simulink model "simTwoLinkFTC"  (R2014b)
settings: Solver=ode45  StartTime=0.0  StopTime=tof  FixedStep=dt  MaxStep=dtmax  RelTol=1e-3
values from neighbouring files (symbols this model uses):
  alpha = 1    [robotArmWith2Links.m]    (also in threeLinkFTC.m; twoLinkFTC.m; twoLinkFTCwAdaptive.m)
  Ar = [0 5; -30 -30]    [robotArmWith2Links.m]    (also in threeLinkFTC.m = [0 1; -5 -5]; twoLinkFTC.m = [0 10; -40 -40]; twoLinkFTCwAdaptive.m = [0 5; -250 -250])
  Arm1 = [0 1; -wn^2 -2*ksi*wn]    [robotArmWith2Links.m]    (also in threeLinkFTC.m; twoLinkFTC.m; twoLinkFTCwAdaptive.m)
  As = zeros(nofstates,nofstates)    [threeLinkFTC.m]    (also in twoLinkFDIbasisComparison.m; twoLinkFTC.m; twoLinkFTCwAdaptive.m)
  Brm1 = [0 wn^2]'    [robotArmWith2Links.m]    (also in threeLinkFTC.m; twoLinkFTC.m; twoLinkFTCwAdaptive.m)
  c1 = 0    [robotArmWith2Links.m]    (also in twoLinkFDIbasisComparison.m = 1; twoLinkFTC.m; twoLinkFTCwAdaptive.m)
  c2 = 0    [robotArmWith2Links.m]    (also in twoLinkFDIbasisComparison.m = 1; twoLinkFTC.m; twoLinkFTCwAdaptive.m)
  Dhat0 = zeros(6,1)    [threeLinkFTC.m]    (also in twoLinkFDIbasisComparison.m = zeros(4,1); twoLinkFTC.m = zeros(4,1); twoLinkFTCwAdaptive.m = zeros(4,1))
  Dlimit = 10    [threeLinkFTC.m]    (also in twoLinkFTC.m; twoLinkFTCwAdaptive.m)
  dtFc = 1*dtmax    (= 0.001)    [threeLinkFTC.m]    (also in twoLinkFDIbasisComparison.m; twoLinkFTC.m; twoLinkFTCwAdaptive.m)
  epsilon = 0.5    [robotArmWith2Links.m]    (also in threeLinkFTC.m; twoLinkFTC.m; twoLinkFTCwAdaptive.m)
  epsilontheta = 0.01    [threeLinkFTC.m]    (also in twoLinkFDIbasisComparison.m; twoLinkFTC.m; twoLinkFTCwAdaptive.m)
  faultyArm = 3    [threeLinkFTC.m]    (also in twoLinkFDIbasisComparison.m = 2; twoLinkFTC.m = 2; twoLinkFTCwAdaptive.m = 1)
  FDstart = 0.5    [threeLinkFTC.m]    (also in twoLinkFTC.m; twoLinkFTCwAdaptive.m)
  fmPosition = [0 90 -45]'*pi/180    [threeLinkFTC.m]    (also in twoLinkFTC.m = [90 0]'*pi/180; twoLinkFTCwAdaptive.m = [90 0]'*pi/180)
  g = 9.81    [robotArmWith2Links.m]    (also in threeLinkFTC.m; twoLinkFDIbasisComparison.m; twoLinkFTC.m; twoLinkFTCwAdaptive.m)
  GammaW = 1000    [threeLinkFTC.m]    (also in twoLinkFDIbasisComparison.m; twoLinkFTC.m; twoLinkFTCwAdaptive.m)
  I1 = 8.33e-2    (= 0.0833)    [robotArmWith2Links.m]    (also in threeLinkFTC.m = 0.0833333333333; twoLinkFDIbasisComparison.m = 0.0833333333333; twoLinkFTC.m = 0.0833333333333; twoLinkFTCwAdaptive.m = 0.0833333333333)
  I2 = 8.33e-2    (= 0.0833)    [robotArmWith2Links.m]    (also in threeLinkFTC.m = 0.0833333333333; twoLinkFDIbasisComparison.m = 0.0833333333333; twoLinkFTC.m = 0.0833333333333; twoLinkFTCwAdaptive.m = 0.0833333333333)
  ifault = 2    [threeLinkFTC.m]    (also in twoLinkFDIbasisComparison.m; twoLinkFTC.m; twoLinkFTCwAdaptive.m)
  K1 = 2*wn*ksi    (= 87.9645943005)    [robotArmWith2Links.m]    (also in threeLinkFTC.m = 8.79645943005; twoLinkFTC.m; twoLinkFTCwAdaptive.m = 43.9822971503)
  K2 = wn^2    (= 986.960440109)    [robotArmWith2Links.m]    (also in threeLinkFTC.m = 39.4784176044; twoLinkFTC.m; twoLinkFTCwAdaptive.m)
  Kp = wn^2    (= 157.913670417)    [threeLinkFTC.m]    (also in twoLinkFDIbasisComparison.m = 3947.84176044; twoLinkFTC.m = 3947.84176044; twoLinkFTCwAdaptive.m = 3947.84176044)
  Kv = 2*ksi*wn    (= 17.5929188601)    [threeLinkFTC.m]    (also in twoLinkFDIbasisComparison.m = 125.663706144; twoLinkFTC.m = 125.663706144; twoLinkFTCwAdaptive.m = 125.663706144)
  l1 = 1    [robotArmWith2Links.m]    (also in threeLinkFTC.m; twoLinkFDIbasisComparison.m; twoLinkFTC.m; twoLinkFTCwAdaptive.m)
  l2 = 1    [robotArmWith2Links.m]    (also in threeLinkFTC.m; twoLinkFDIbasisComparison.m; twoLinkFTC.m; twoLinkFTCwAdaptive.m)
  lc1 = l1/2    (= 0.5)    [robotArmWith2Links.m]    (also in threeLinkFTC.m; twoLinkFDIbasisComparison.m; twoLinkFTC.m; twoLinkFTCwAdaptive.m)
  lc2 = l2/2    (= 0.5)    [robotArmWith2Links.m]    (also in threeLinkFTC.m; twoLinkFDIbasisComparison.m; twoLinkFTC.m; twoLinkFTCwAdaptive.m)
  m1 = 1    [robotArmWith2Links.m]    (also in threeLinkFTC.m; twoLinkFDIbasisComparison.m; twoLinkFTC.m; twoLinkFTCwAdaptive.m)
  m2 = 1    [robotArmWith2Links.m]    (also in threeLinkFTC.m; twoLinkFDIbasisComparison.m; twoLinkFTC.m; twoLinkFTCwAdaptive.m)
  nCheby = 4    [threeLinkFTC.m]    (also in twoLinkFDIbasisComparison.m; twoLinkFTC.m; twoLinkFTCwAdaptive.m)
  Ps = lyap(As(4:6,4:6)',Q)    [threeLinkFTC.m]    (also in twoLinkFDIbasisComparison.m = lyap(As(3:4,3:4)',Q); twoLinkFTC.m = lyap(As(3:4,3:4)',Q); twoLinkFTCwAdaptive.m = lyap(As(3:4,3:4)',Q))
  q0 = [80 20]'*pi/180    [robotArmWith2Links.m]    (also in threeLinkFTC.m = [90 0 0]'*pi/180; twoLinkFDIbasisComparison.m = [90 0]'*pi/180; twoLinkFTC.m = [90 0]'*pi/180; twoLinkFTCwAdaptive.m = [90 0]'*pi/180)
  qdot0 = [0 0]'    [robotArmWith2Links.m]    (also in threeLinkFTC.m = [0 0 0]'*pi/180; twoLinkFDIbasisComparison.m = [0 0]'*pi/180; twoLinkFTC.m = [0 0]'*pi/180; twoLinkFTCwAdaptive.m = [0 0]'*pi/180)
  r0 = [0 0]'    [robotArmWith2Links.m]    (also in threeLinkFTC.m; twoLinkFTC.m; twoLinkFTCwAdaptive.m)
  rmax = inf*[50*pi/180 inf]'    [robotArmWith2Links.m]    (also in threeLinkFTC.m; twoLinkFTC.m; twoLinkFTCwAdaptive.m)
  rmin = -rmax    [robotArmWith2Links.m]    (also in threeLinkFTC.m; twoLinkFTC.m; twoLinkFTCwAdaptive.m)
  tfault = 5    [threeLinkFTC.m]    (also in twoLinkFDIbasisComparison.m; twoLinkFTC.m; twoLinkFTCwAdaptive.m = 1)
  visualFlag = 0    [robotArmWith2Links.m]    (also in twoLinkFDIbasisComparison.m; twoLinkFTC.m; twoLinkFTCwAdaptive.m)
  visualizationDataFlag = 1    [robotArmWith2Links.m]    (also in twoLinkFDIbasisComparison.m; twoLinkFTC.m; twoLinkFTCwAdaptive.m)
  W0 = 0    [threeLinkFTC.m]    (also in twoLinkFDIbasisComparison.m; twoLinkFTC.m; twoLinkFTCwAdaptive.m)
  Wbnd = 1000    [threeLinkFTC.m]    (also in twoLinkFDIbasisComparison.m; twoLinkFTC.m; twoLinkFTCwAdaptive.m)
  xhat0 = [q0 ; qdot0]    [threeLinkFTC.m]    (also in twoLinkFDIbasisComparison.m; twoLinkFTC.m; twoLinkFTCwAdaptive.m)
undefined symbols (not defined in the file or in its folder): Intmax, Intmin, twolinkplot
libraries: simulink x6, vrlib x2, dspbuff3 x1
(part 2 of 2)

== system simTwoLinkFTC/System/System Parameters/Energy Calculation ==
  q : Inport
  qdot : Inport  Port=2
  H : Inport  Port=3
  Constant : Constant  Value=l1  VectorParams1D=off
  Constant1 : Constant  Value=l2  VectorParams1D=off
  Demux : Demux  Outputs=2
  Gain : Gain  Gain=1/2
  Gain1 : Gain  Gain=0.5
  Gain5 : Gain  Gain=0.5*m1*g
  Gain6 : Gain  Gain=m2*g
  Math Function : Math  Operator=transpose  SaturateOnIntegerOverflow=on
  Product1 : Product  RndMeth=Zero
  Product3 : Product  RndMeth=Zero
  Product5 : Product  Inputs=3  Multiplication=Matrix(*)  RndMeth=Zero
  Sum of Elements : Sum  Inputs=+
  Sum1 : Sum
  Sum2 : Sum
  Sum3 : Sum
  Terminator4 : Terminator
  Trigonometric Function : Trigonometry
  Trigonometric Function2 : Trigonometry
  U : Outport
  T : Outport  Port=2
  E : Outport  Port=3
  wires:
  [q] -> Trigonometric Function/1, Sum of Elements/1
  Trigonometric Function/1 -> Demux/1
  Demux/1 -> [s1]
  Demux/2 -> Terminator4/1
  Sum of Elements/1 -> Trigonometric Function2/1
  Trigonometric Function2/1 -> [s12]
  [qdot] -> Math Function/1
  Math Function/1 -> Product5/1
  [H] -> Product5/2
  [qdot] -> Product5/3
  Product5/1 -> Gain/1
  [l1sintht1] -> Gain5/1
  Gain/1 -> [T]
  [l1sintht1] -> Sum1/1
  [l2sintht12] -> Gain1/1
  Gain5/1 -> Sum3/1
  Gain6/1 -> Sum3/2
  [T] -> Sum2/1
  [U] -> Sum2/2
  q/1 -> [q]
  qdot/1 -> [qdot]
  Sum2/1 -> E/1  "E"
  [U] -> U/1  "U"
  [T] -> T/1  "T"
  Constant/1 -> Product1/1
  [s1] -> Product1/2
  Product1/1 -> [l1sintht1]
  Constant1/1 -> Product3/1
  [s12] -> Product3/2
  Product3/1 -> [l2sintht12]
  Gain1/1 -> Sum1/2
  Sum1/1 -> Gain6/1
  Sum3/1 -> [U]
  H/1 -> [H]

== system simTwoLinkFTC/System/System Parameters/get Plant Parameters ==
  H : Inport
  C : Inport  Port=2
  G : Inport  Port=3
  qdot : Inport  Port=4
  {1,5,7,11} (4 alike) : Selector  NumberOfDimensions=2  InputPortWidth=3  IndexOptions=Index vector (dialog),Index vector (dialog)  Indices=1,1  OutputSizes=1,1
  12 : Selector  NumberOfDimensions=2  InputPortWidth=3  IndexOptions=Index vector (dialog),Index vector (dialog)  Indices=1,2  OutputSizes=1,1
  2 : Selector  NumberOfDimensions=2  InputPortWidth=3  IndexOptions=Index vector (dialog),Index vector (dialog)  Indices=1,2  OutputSizes=1,1
  {3,6,8,21} (4 alike) : Selector  NumberOfDimensions=2  InputPortWidth=3  IndexOptions=Index vector (dialog),Index vector (dialog)  Indices=2,1  OutputSizes=1,1
  22 : Selector  NumberOfDimensions=2  InputPortWidth=3  IndexOptions=Index vector (dialog),Index vector (dialog)  Indices=2,2  OutputSizes=1,1
  4 : Selector  NumberOfDimensions=2  InputPortWidth=3  IndexOptions=Index vector (dialog),Index vector (dialog)  Indices=2,2  OutputSizes=1,1
  Bus Creator : BusCreator  Inputs=15
  Product5 : Product  Multiplication=Matrix(*)  RndMeth=Zero
  Sum of Elements1 : Sum
  busData : Outport
  wires:
  2/1 -> Bus Creator/9  "C12"
  21/1 -> Bus Creator/6  "H21"
  22/1 -> Bus Creator/7  "H22"
  4/1 -> Bus Creator/11  "C22"
  6/1 -> Bus Creator/13  "G_2"
  1/1 -> Bus Creator/8  "C11"
  5/1 -> Bus Creator/12  "G_1"
  12/1 -> Bus Creator/5  "H12"
  3/1 -> Bus Creator/10  "C21"
  11/1 -> Bus Creator/4  "H11"
  [H] -> 11/1, 12/1, 21/1, 22/1
  [C] -> 1/1, 2/1, 4/1, 3/1
  [G] -> 6/1, 5/1
  [C] -> Product5/1
  [qdot] -> Product5/2
  Product5/1 -> Sum of Elements1/1
  [G] -> Sum of Elements1/2
  Sum of Elements1/1 -> 7/1, 8/1
  7/1 -> Bus Creator/14  "phi1"
  8/1 -> Bus Creator/15  "phi2"
  [G] -> Bus Creator/3
  Bus Creator/1 -> busData/1
  [C] -> Bus Creator/2
  [H] -> Bus Creator/1
  H/1 -> [H]  "H"
  C/1 -> [C]  "C"
  G/1 -> [G]  "G"
  qdot/1 -> [qdot]

== system simTwoLinkFTC/System/System Parameters/getC ==
  s2 : Inport
  q1dot : Inport  Port=2
  q2dot : Inport  Port=3
  m2 : Inport  Port=4
  Add : Sum
  Constant2 : Constant  Value=c2  VectorParams1D=off
  Constant3 : Constant  Value=c1  VectorParams1D=off
  Gain4 : Gain  Gain=l1*lc2
  Gain6 : Gain  Gain=-1
  Gain7 : Gain  Gain=-1
  Matrix Concatenate : Concatenate  Mode=Multidimensional array  ConcatenateDimension=2
  Matrix Concatenate1 : Concatenate  Mode=Multidimensional array  ConcatenateDimension=2
  Matrix Concatenate2 : Concatenate  Mode=Multidimensional array
  Product{,8..10} (4 alike) : Product  RndMeth=Zero
  Sum4 : Sum
  C : Outport
  wires:
  s2/1 -> [s2]
  q1dot/1 -> [q1dot]
  q2dot/1 -> [q2dot]
  [C] -> C/1
  [m2] -> Gain4/1
  Gain4/1 -> Product/1
  [s2] -> Product/2
  Product/1 -> [h]
  [h] -> Gain6/1
  [h] -> Gain7/1
  Sum4/1 -> Product10/1
  Gain7/1 -> Product10/2
  Product10/1 -> [C12]
  [q2dot] -> Sum4/2
  Constant2/1 -> [C22]
  [h] -> Product8/2
  [q1dot] -> Product8/1
  Product8/1 -> [C21]
  Gain6/1 -> Product9/2
  [q2dot] -> Product9/1
  [q1dot] -> Sum4/1
  Matrix Concatenate2/1 -> [C]
  [C22] -> Matrix Concatenate1/2
  [C21] -> Matrix Concatenate1/1
  Matrix Concatenate1/1 -> Matrix Concatenate2/2
  Matrix Concatenate/1 -> Matrix Concatenate2/1
  [C12] -> Matrix Concatenate/2
  [C11] -> Matrix Concatenate/1
  Product9/1 -> Add/1
  Constant3/1 -> Add/2
  Add/1 -> [C11]
  m2/1 -> [m2]

== system simTwoLinkFTC/System/System Parameters/getG ==
  c1 : Inport
  c12 : Inport  Port=2
  m1 : Inport  Port=3
  m2 : Inport  Port=4
  Add1 : Sum
  Add2 : Sum
  Gain10 : Gain  Gain=lc2
  Gain11 : Gain  Gain=g
  Gain5 : Gain  Gain=lc1
  Gain6 : Gain  Gain=l1
  Gain7 : Gain  Gain=g
  Gain8 : Gain  Gain=lc2
  Gain9 : Gain  Gain=g
  Matrix Concatenate2 : Concatenate  Mode=Multidimensional array
  Product1 : Product  RndMeth=Zero
  Product2 : Product  RndMeth=Zero
  Product3 : Product  RndMeth=Zero
  G : Outport
  wires:
  c12/1 -> [c12]
  c1/1 -> [c1]
  Matrix Concatenate2/1 -> G/1
  [G11] -> Matrix Concatenate2/1
  [G21] -> Matrix Concatenate2/2
  [m1] -> Gain5/1
  Gain5/1 -> Add1/1
  [m2] -> Gain6/1
  Gain6/1 -> Add1/2
  Add1/1 -> Gain7/1
  Gain7/1 -> Product1/1
  [c1] -> Product1/2
  [m2] -> Gain8/1
  Gain8/1 -> Gain9/1
  Gain9/1 -> Product2/1
  [c12] -> Product2/2
  Product1/1 -> Add2/1
  Product2/1 -> Add2/2
  Add2/1 -> [G11]
  [m2] -> Gain10/1
  Gain10/1 -> Gain11/1
  Gain11/1 -> Product3/1
  [c12] -> Product3/2
  Product3/1 -> [G21]
  m1/1 -> [m1]
  m2/1 -> [m2]

== system simTwoLinkFTC/System/System Parameters/getH ==
  c2 : Inport
  m1 : Inport  Port=2
  m2 : Inport  Port=3
  I1 : Inport  Port=4
  I2 : Inport  Port=5
  Gain : Gain  Gain=2
  Gain1 : Gain  Gain=lc2^2
  Gain4 : Gain  Gain=l1*lc2
  Gain5 : Gain  Gain=lc1^2
  Gain6 : Gain  Gain=l1^2+lc2^2
  Gain7 : Gain  Gain=lc2^2
  Matrix Concatenate : Concatenate  Mode=Multidimensional array  ConcatenateDimension=2
  Matrix Concatenate1 : Concatenate  Mode=Multidimensional array  ConcatenateDimension=2
  Matrix Concatenate2 : Concatenate  Mode=Multidimensional array
  Product : Product  RndMeth=Zero
  Sum : Sum  Inputs=+++++
  Sum1 : Sum  Inputs=+++
  Sum2 : Sum
  H : Outport
  wires:
  [H11] -> Matrix Concatenate/1
  [H12] -> Matrix Concatenate/2
  Matrix Concatenate/1 -> Matrix Concatenate2/1
  Matrix Concatenate1/1 -> Matrix Concatenate2/2
  [H21] -> Matrix Concatenate1/1
  [H22] -> Matrix Concatenate1/2
  Matrix Concatenate2/1 -> H/1
  c2/1 -> [c2]
  Sum/1 -> [H11]
  Sum1/1 -> [H12], [H21]
  [m2] -> Gain4/1
  Gain4/1 -> Product/1
  [c2] -> Product/2
  Product/1 -> [a]
  [m1] -> Gain5/1
  [m2] -> Gain6/1
  [I1] -> Sum/1
  [I2] -> Sum/2
  Gain5/1 -> Sum/3
  [a] -> Gain/1
  Gain6/1 -> Sum/4
  Gain/1 -> Sum/5
  [m2] -> Gain7/1
  [I2] -> Sum1/1
  Gain7/1 -> Sum1/2
  [a] -> Sum1/3
  [m2] -> Gain1/1
  [I2] -> Sum2/1
  Gain1/1 -> Sum2/2
  Sum2/1 -> [H22]
  m1/1 -> [m1]
  m2/1 -> [m2]
  I1/1 -> [I1]
  I2/1 -> [I2]

== system simTwoLinkFTC/System/System Parameters/getH1 ==
  c2 : Inport
  m1 : Inport  Port=2
  m2 : Inport  Port=3
  I1 : Inport  Port=4
  I2 : Inport  Port=5
  Gain : Gain  Gain=2
  Gain1 : Gain  Gain=lc2^2
  Gain4 : Gain  Gain=l1*lc2
  Gain5 : Gain  Gain=lc1^2
  Gain6 : Gain  Gain=l1^2+lc2^2
  Gain7 : Gain  Gain=lc2^2
  Matrix Concatenate : Concatenate  Mode=Multidimensional array  ConcatenateDimension=2
  Matrix Concatenate1 : Concatenate  Mode=Multidimensional array  ConcatenateDimension=2
  Matrix Concatenate2 : Concatenate  Mode=Multidimensional array
  Product : Product  RndMeth=Zero
  Sum : Sum  Inputs=+++++
  Sum1 : Sum  Inputs=+++
  Sum2 : Sum
  H : Outport
  wires:
  [H11] -> Matrix Concatenate/1
  [H12] -> Matrix Concatenate/2
  Matrix Concatenate/1 -> Matrix Concatenate2/1
  Matrix Concatenate1/1 -> Matrix Concatenate2/2
  [H21] -> Matrix Concatenate1/1
  [H22] -> Matrix Concatenate1/2
  Matrix Concatenate2/1 -> H/1
  c2/1 -> [c2]
  Sum/1 -> [H11]
  Sum1/1 -> [H12], [H21]
  [m2] -> Gain4/1
  Gain4/1 -> Product/1
  [c2] -> Product/2
  Product/1 -> [a]
  [m1] -> Gain5/1
  [m2] -> Gain6/1
  [I1] -> Sum/1
  [I2] -> Sum/2
  Gain5/1 -> Sum/3
  [a] -> Gain/1
  Gain6/1 -> Sum/4
  Gain/1 -> Sum/5
  [m2] -> Gain7/1
  [I2] -> Sum1/1
  Gain7/1 -> Sum1/2
  [a] -> Sum1/3
  [m2] -> Gain1/1
  [I2] -> Sum2/1
  Gain1/1 -> Sum2/2
  Sum2/1 -> [H22]
  m1/1 -> [m1]
  m2/1 -> [m2]
  I1/1 -> [I1]
  I2/1 -> [I2]

== system simTwoLinkFTC/System/System Parameters/getMass ==
  Constant : Constant  Value=m1
  Constant1 : Constant  Value=m2
  Constant5 : Constant  Value=I1
  Constant6 : Constant  Value=I2
  m1 : Outport
  m2 : Outport  Port=2
  I1 : Outport  Port=3
  I2 : Outport  Port=4
  wires:
  [m1] -> m1/1  "m1"
  [m2] -> m2/1  "m2"
  [I1] -> I1/1  "I1"
  [I2] -> I2/1  "I2"
  Constant5/1 -> [I1]
  Constant/1 -> [m1]
  Constant1/1 -> [m2]
  Constant6/1 -> [I2]

== system simTwoLinkFTC/Controller/Disturbance Estimator/getDisturbance/Chebyshev Basis Functions ==
  x : Inport
  tau : Inport  Port=2
  Chebyshev Polynomail Value Calculation : Subsystem  TreatAsAtomicUnit=on
  Demux : Demux
  Mux : Mux
  Reshape1 : Reshape  OutputDimensionality=Column vector (2-D)
  Reshape2 : Reshape  OutputDimensionality=Column vector (2-D)
  Terminator1 : Terminator
  Tn : Outport
  wires:
  [Tn] -> Tn/1
  [z] -> Chebyshev Polynomail Value Calculation/1(x)
  Chebyshev Polynomail Value Calculation/1(chebyPol) -> Reshape2/1
  Reshape2/1 -> [Tn]
  tau/1 -> Terminator1/1
  x/1 -> [x]
  [x] -> Demux/1
  Demux/1 -> [q1]
  Demux/2 -> [q2]
  Demux/3 -> [q1dot]
  Demux/4 -> [q2dot]
  Mux/1 -> Reshape1/1
  Reshape1/1 -> [z]
  [q1] -> Mux/1
  [q2] -> Mux/2
  [q1dot] -> Mux/3
  [q2dot] -> Mux/4

== system simTwoLinkFTC/Controller/Disturbance Estimator/getDisturbance/Custom Basis Functions ==
  x : Inport
  tau : Inport  Port=2
  Add : Sum
  Constant : Constant
  Demux : Demux
  Math Function : Math  Operator=square  SaturateOnIntegerOverflow=on
  Math Function1 : Math  Operator=square  SaturateOnIntegerOverflow=on
  Mux : Mux  Inputs=7
  Product{1..4} (4 alike) : Product  RndMeth=Zero
  Reshape : Reshape  OutputDimensionality=Column vector (2-D)
  Terminator1 : Terminator
  Trigonometric Function : Trigonometry  Operator=cos
  Trigonometric Function1 : Trigonometry  Operator=cos
  Trigonometric Function{2..5} (4 alike) : Trigonometry
  psiz : Outport
  wires:
  [psiz] -> psiz/1
  Constant/1 -> Mux/1
  Mux/1 -> Reshape/1
  Reshape/1 -> [psiz]
  tau/1 -> Terminator1/1
  x/1 -> [x]
  [x] -> Demux/1
  Demux/1 -> [q1]
  Demux/2 -> [q2]
  Demux/3 -> [q1dot]
  Demux/4 -> [q2dot]
  [q1] -> Trigonometric Function/1
  Trigonometric Function/1 -> Mux/2
  [q1] -> Add/1
  [q2] -> Add/2
  Add/1 -> Trigonometric Function1/1
  Trigonometric Function1/1 -> Mux/3
  [q2] -> Trigonometric Function2/1
  Trigonometric Function2/1 -> Product1/1
  [q1dot] -> Product1/2
  Product1/1 -> Mux/4
  [q2] -> Trigonometric Function3/1
  Trigonometric Function3/1 -> Product2/1
  [q2dot] -> Product2/2
  Product2/1 -> Mux/5
  [q2] -> Trigonometric Function4/1
  Trigonometric Function4/1 -> Product3/1
  [q1dot] -> Math Function/1
  Math Function/1 -> Product3/2
  Product3/1 -> Mux/6
  [q2] -> Trigonometric Function5/1
  Trigonometric Function5/1 -> Product4/1
  [q2dot] -> Math Function1/1
  Math Function1/1 -> Product4/2
  Product4/1 -> Mux/7

== system simTwoLinkFTC/Controller/Disturbance Estimator/getDisturbance/getDhat ==
  psiz : Inport
  es : Inport  Port=2
  Bus Creator : BusCreator  Inputs=2
  Math Function : Math  Operator=transpose  SaturateOnIntegerOverflow=on
  Math Function1 : Math  Operator=transpose  SaturateOnIntegerOverflow=on
  Reshape : Reshape  OutputDimensionality=Column vector (2-D)
  Selector : Selector  NumberOfDimensions=2  InputPortWidth=3  IndexOptions=Select all,Index vector (dialog)  Indices=[1 3],1  OutputSizes=1,1
  Selector1 : Selector  NumberOfDimensions=2  InputPortWidth=3  IndexOptions=Select all,Index vector (dialog)  Indices=[1 3],2  OutputSizes=1,1
  Terminator1 : Terminator
  Vector Concatenate : Concatenate
  adaptiveGain : Subsystem  TreatAsAtomicUnit=on
  getW1 : Subsystem
  getW2 : Subsystem
  Dhat : Outport
  wires:
  es/1 -> [es]  "es"
  adaptiveGain/1(Wintegrand) -> [Wint]  "Wint"
  [Dhat] -> Dhat/1  "Dhat"
  psiz/1 -> [psiz]  "psiz"
  [es] -> adaptiveGain/2(es)
  [psiz] -> adaptiveGain/1(psi(z))
  [psiz] -> getW1/2(psiz)
  Selector/1 -> getW1/1(Wint)
  Vector Concatenate/1 -> Reshape/1
  [psiz] -> getW2/2(psiz)
  Selector1/1 -> getW2/1(Wint)
  Reshape/1 -> [Dhat]
  Bus Creator/1 -> Terminator1/1  "W"
  getW2/2(WTpsi) -> Vector Concatenate/2
  getW1/2(WTpsi) -> Vector Concatenate/1
  getW1/1(W) -> Math Function/1
  getW2/1(W) -> Math Function1/1
  [Wint] -> Selector1/1, Selector/1
  Math Function/1 -> Bus Creator/1  "W1"
  Math Function1/1 -> Bus Creator/2  "W2"

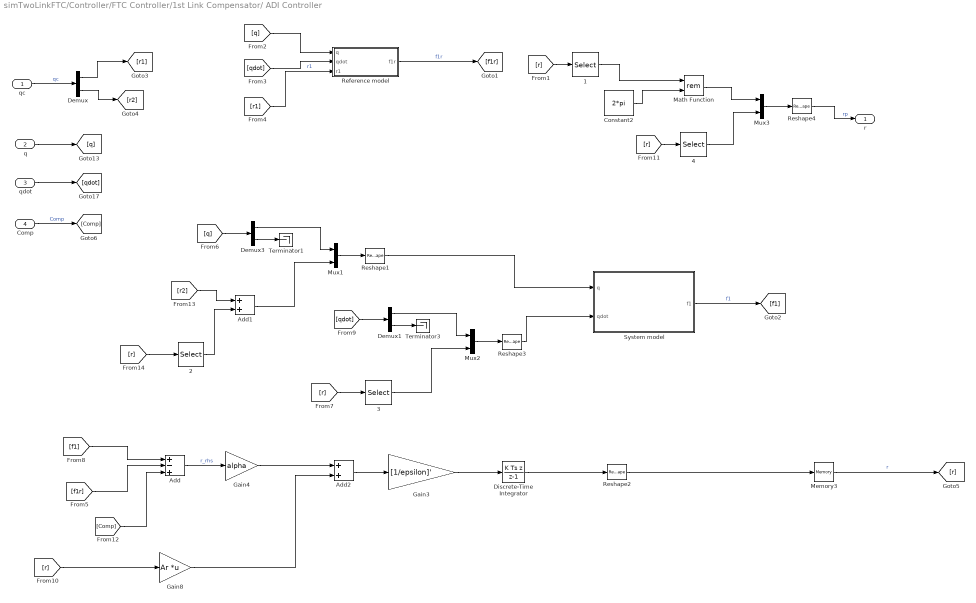
== system simTwoLinkFTC/Controller/FTC Controller/1st Link Compensator/ ADI Controller ==
  qc : Inport
  q : Inport  Port=2
  qdot : Inport  Port=3
  Comp : Inport  Port=4
  1 : Selector  NumberOfDimensions=2  InputPortWidth=3  IndexOptions=Index vector (dialog),Index vector (dialog)  Indices=1,1  OutputSizes=1,1
  2 : Selector  NumberOfDimensions=2  InputPortWidth=3  IndexOptions=Index vector (dialog),Index vector (dialog)  Indices=1,1  OutputSizes=1,1
  3 : Selector  NumberOfDimensions=2  InputPortWidth=3  IndexOptions=Index vector (dialog),Index vector (dialog)  Indices=2,1  OutputSizes=1,1
  4 : Selector  NumberOfDimensions=2  InputPortWidth=3  IndexOptions=Index vector (dialog),Index vector (dialog)  Indices=2,1  OutputSizes=1,1
  Add : Sum  Inputs=+-+
  Add1 : Sum
  Add2 : Sum
  Constant2 : Constant  Value=2*pi
  Demux : Demux  Outputs=2
  Demux1 : Demux  Outputs=2
  Demux3 : Demux  Outputs=2
  Discrete-Time Integrator : DiscreteIntegrator  IntegratorMethod=Integration: Backward Euler  InitialCondition=r0  InitialConditionSetting=State (most efficient)  SampleTime=-1  LimitOutput=on  UpperSaturationLimit=rmax  LowerSaturationLimit=rmin
  Gain3 : Gain  Gain=[1/epsilon]'
  Gain4 : Gain  Gain=alpha
  Gain8 : Gain  Gain=Ar  Multiplication=Matrix(K*u)
  Math Function : Math  Operator=rem  SaturateOnIntegerOverflow=on
  Memory3 : Memory  X0=r0  InheritSampleTime=on  LinearizeMemory=on  LinearizeAsDelay=on
  Mux1 : Mux  Inputs=2
  Mux2 : Mux  Inputs=2
  Mux3 : Mux  Inputs=2
  Reference model : Subsystem  TreatAsAtomicUnit=on
  Reshape{1..4} (4 alike) : Reshape  OutputDimensionality=Column vector (2-D)
  System model : Subsystem  TreatAsAtomicUnit=on
  Terminator1 : Terminator
  Terminator3 : Terminator
  r : Outport
  wires:
  qc/1 -> Demux/1  "qc"
  Add/1 -> Gain4/1  "r_rhs"
  [f1] -> Add/1
  [f1r] -> Add/2
  Gain4/1 -> Add2/1
  Add2/1 -> Gain3/1
  q/1 -> [q]
  qdot/1 -> [qdot]
  [qdot] -> Reference model/2(qdot)
  [q] -> Reference model/1(q)
  [r1] -> Reference model/3(r1)  "r1"
  Reference model/1(f1r) -> [f1r]  "f1r"
  System model/1(f1) -> [f1]  "f1"
  Gain8/1 -> Add2/2
  Reshape3/1 -> System model/2(qdot)
  Demux3/1 -> Mux1/1
  Mux1/1 -> Reshape1/1
  Reshape1/1 -> System model/1(q)
  [q] -> Demux3/1
  Demux3/2 -> Terminator1/1
  [r2] -> Add1/1
  Add1/1 -> Mux1/2
  Memory3/1 -> [r]  "r"
  Constant2/1 -> Math Function/2
  [r] -> 1/1
  Gain3/1 -> Discrete-Time Integrator/1
  Discrete-Time Integrator/1 -> Reshape2/1
  Demux/1 -> [r1]
  Demux/2 -> [r2]
  [r] -> 2/1
  2/1 -> Add1/2
  Demux1/1 -> Mux2/1
  Mux2/1 -> Reshape3/1
  [qdot] -> Demux1/1
  Demux1/2 -> Terminator3/1
  3/1 -> Mux2/2
  [r] -> 3/1
  1/1 -> Math Function/1
  [r] -> Gain8/1
  Mux3/1 -> Reshape4/1
  Reshape4/1 -> r/1  "rp"
  [r] -> 4/1
  Comp/1 -> [Comp]  "Comp"
  [Comp] -> Add/3
  Math Function/1 -> Mux3/1
  4/1 -> Mux3/2
  Reshape2/1 -> Memory3/1

== system simTwoLinkFTC/Controller/FTC Controller/1st Link Compensator/Partial FBL q2 Controller ==
  qc : Inport
  qcdot : Inport  Port=2
  q : Inport  Port=3
  qdot : Inport  Port=4
  H : Inport  Port=5
  C : Inport  Port=6
  G : Inport  Port=7
  Collocated q2 Controller : Subsystem  TreatAsAtomicUnit=on
  Demux{,1..3} (4 alike) : Demux  Outputs=2
  Terminator{1..4} (4 alike) : Terminator
  Torque calculation : Subsystem  TreatAsAtomicUnit=on
  tau : Outport
  v : Outport  Port=2
  wires:
  [q] -> Collocated q2 Controller/3(q)
  Collocated q2 Controller/1(v) -> [v]  "v"
  C/1 -> [C]
  H/1 -> [H]
  qc/1 -> Demux/1
  Demux/1 -> Terminator2/1
  Demux/2 -> [r]
  G/1 -> [G]
  Torque calculation/1(tau) -> [tau]
  [v] -> Torque calculation/1(v)
  [H] -> Torque calculation/2(H)
  [C] -> Torque calculation/3(C)
  [G] -> Torque calculation/4(G)
  [r] -> Collocated q2 Controller/1(r)
  q/1 -> Demux1/1
  Demux1/1 -> Terminator1/1
  Demux1/2 -> [q]
  [qdot] -> Torque calculation/5(qdot)
  qdot/1 -> [qdot]
  [qdot] -> Demux2/1
  Demux2/2 -> Collocated q2 Controller/4(qdot)
  Demux2/1 -> Terminator3/1
  [v] -> v/1
  qcdot/1 -> Demux3/1
  Demux3/1 -> Terminator4/1
  Demux3/2 -> [rdot]
  [rdot] -> Collocated q2 Controller/2(rdot)
  [tau] -> tau/1

== system simTwoLinkFTC/Controller/Disturbance Estimator/getDisturbance/Chebyshev Basis Functions/Chebyshev Polynomail Value Calculation ==
  x : Inport
  Delay Line : dspbuff3/Delay Line  siz=nCheby  ic=zeros(nCheby,1)  directfeed=on  enable_output=off  hold_output=off  TreatMby1Signals=M channels (this choice will be removed - see release notes)
  For Iterator : ForIterator  IterationLimit=nCheby
  Frame Conversion : FrameConversion  OutFrame=Sample-based
  If : If  IfExpression=u1 > 2
  If Action Subsystem : Subsystem  TreatAsAtomicUnit=on
  If Action Subsystem1 : Subsystem  TreatAsAtomicUnit=on
  Memory : Memory  InheritSampleTime=on  LinearizeMemory=on  LinearizeAsDelay=on
  Merge : Merge
  Reshape : Reshape  OutputDimensionality=Column vector (2-D)
  chebyPol : Outport
  wires:
  For Iterator/1 -> [N]
  x/1 -> [x]
  [N] -> If/1
  If/1 -> If Action Subsystem/Action
  If/2 -> If Action Subsystem1/Action
  [N] -> If Action Subsystem1/2(N)
  [x] -> If Action Subsystem1/1(x)
  [x] -> If Action Subsystem/1(x)
  If Action Subsystem/1(polyval) -> Merge/1
  If Action Subsystem1/1(polval) -> Merge/2
  Merge/1 -> [polyval]
  [polyval] -> Delay Line/1
  Delay Line/1 -> Frame Conversion/1
  Reshape/1 -> [polyvals]
  [polyvals] -> Memory/1
  [polyvals] -> chebyPol/1  "chebyPol"
  Frame Conversion/1 -> Reshape/1
  Memory/1 -> If Action Subsystem/2(polyvals)

== system simTwoLinkFTC/Controller/Disturbance Estimator/getDisturbance/getDhat/adaptiveGain ==
  psi(z) : Inport
  es : Inport  Port=2
  Gain1 : Gain  Gain=-1
  Math Function : Math  Operator=transpose  SaturateOnIntegerOverflow=on
  P : Constant  Value=Ps  VectorParams1D=off
  Product1 : Product  Multiplication=Matrix(*)  RndMeth=Zero
  Product3 : Product  Multiplication=Matrix(*)  RndMeth=Zero
  Wintegrand : Outport
  wires:
  Product1/1 -> Product3/2
  psi(z)/1 -> Product3/1
  Gain1/1 -> Wintegrand/1
  es/1 -> Math Function/1
  Math Function/1 -> Product1/1
  P/1 -> Product1/2
  Product3/1 -> Gain1/1

== system simTwoLinkFTC/Controller/Disturbance Estimator/getDisturbance/getDhat/getW1 ==
  Wint : Inport
  psiz : Inport  Port=2
  Constant : Constant  Value=Wbnd  VectorParams1D=off
  Constant1 : Constant  Value=epsilontheta
  Discrete-Time Integrator : DiscreteIntegrator  IntegratorMethod=Integration: Trapezoidal  InitialCondition=W0  SampleTime=-1  LimitOutput=on  UpperSaturationLimit=Wbnd  LowerSaturationLimit=-Wbnd
  Gain : Gain  Gain=GammaW
  Math Function : Math  Operator=transpose  SaturateOnIntegerOverflow=on
  Memory4 : Memory  X0=W0  InheritSampleTime=on  LinearizeMemory=on  LinearizeAsDelay=on
  Product : Product  Multiplication=Matrix(*)  RndMeth=Zero
  Projection : Subsystem  TreatAsAtomicUnit=on
  W : Outport
  WTpsi : Outport  Port=2
  wires:
  [WTpsi] -> WTpsi/1
  [Wint] -> Projection/2(y)
  Math Function/1 -> Product/1
  [psiz] -> Product/2
  Discrete-Time Integrator/1 -> Math Function/1, [W], Memory4/1
  Gain/1 -> Discrete-Time Integrator/1
  Projection/1(Proj) -> Gain/1  "WintProj"
  Memory4/1 -> Projection/1(theta)
  Constant/1 -> Projection/3(Thetamax)
  Constant1/1 -> Projection/4(epsilontheta)
  [W] -> W/1
  Wint/1 -> [Wint]
  psiz/1 -> [psiz]
  Product/1 -> [WTpsi]  "WTpsi"

== system simTwoLinkFTC/Controller/Disturbance Estimator/getDisturbance/getDhat/getW2 ==
  Wint : Inport
  psiz : Inport  Port=2
  Constant : Constant  Value=Wbnd  VectorParams1D=off
  Constant1 : Constant  Value=epsilontheta
  Discrete-Time Integrator : DiscreteIntegrator  IntegratorMethod=Integration: Trapezoidal  InitialCondition=W0  SampleTime=-1  LimitOutput=on  UpperSaturationLimit=Wbnd  LowerSaturationLimit=-Wbnd
  Gain : Gain  Gain=GammaW
  Math Function : Math  Operator=transpose  SaturateOnIntegerOverflow=on
  Memory4 : Memory  X0=W0  InheritSampleTime=on  LinearizeMemory=on  LinearizeAsDelay=on
  Product : Product  Multiplication=Matrix(*)  RndMeth=Zero
  Projection : Subsystem  TreatAsAtomicUnit=on
  W : Outport
  WTpsi : Outport  Port=2
  wires:
  Product/1 -> [WTpsi]  "WTpsi"
  psiz/1 -> [psiz]
  Wint/1 -> [Wint]
  [W] -> W/1
  Constant1/1 -> Projection/4(epsilontheta)
  Constant/1 -> Projection/3(Thetamax)
  Memory4/1 -> Projection/1(theta)
  Projection/1(Proj) -> Gain/1  "WintProj"
  Gain/1 -> Discrete-Time Integrator/1
  Discrete-Time Integrator/1 -> Memory4/1, [W], Math Function/1
  [psiz] -> Product/2
  Math Function/1 -> Product/1
  [Wint] -> Projection/2(y)
  [WTpsi] -> WTpsi/1

== system simTwoLinkFTC/Controller/FTC Controller/1st Link Compensator/ ADI Controller/Reference model ==
  q : Inport
  qdot : Inport  Port=2
  r1 : Inport  Port=3
  Add : Sum
  Constant : Constant  Value=Arm1  VectorParams1D=off
  Constant1 : Constant  Value=Brm1  VectorParams1D=off
  Demux2 : Demux  Outputs=2
  Demux3 : Demux  Outputs=2
  Mux : Mux  Inputs=2
  Product1 : Product  Multiplication=Matrix(*)
  Product3 : Product  Multiplication=Matrix(*)
  Reshape : Reshape  OutputDimensionality=Column vector (2-D)
  Terminator4 : Terminator
  Terminator5 : Terminator
  f1r : Outport
  wires:
  qdot/1 -> Demux3/1
  q/1 -> Demux2/1
  Demux3/2 -> [q2dot]
  Demux3/1 -> [q1dot]
  Demux2/2 -> [q2]
  Demux2/1 -> [q1]
  r1/1 -> [r1]
  Constant/1 -> Product3/1
  [f1r] -> f1r/1
  [q2dot] -> Terminator4/1
  [q2] -> Terminator5/1
  [q1dot] -> Mux/2
  [q1] -> Mux/1
  Mux/1 -> Reshape/1
  Reshape/1 -> Product3/2
  Constant1/1 -> Product1/1
  [r1] -> Product1/2
  Product3/1 -> Add/1
  Product1/1 -> Add/2
  Add/1 -> [f1r]

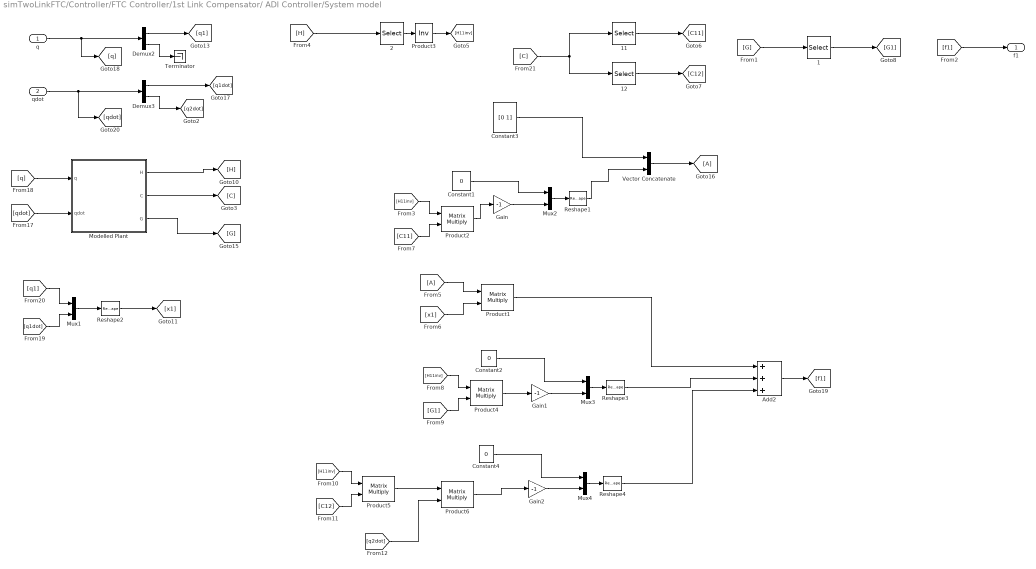
== system simTwoLinkFTC/Controller/FTC Controller/1st Link Compensator/ ADI Controller/System model ==
  q : Inport
  qdot : Inport  Port=2
  1 : Selector  NumberOfDimensions=2  InputPortWidth=3  IndexOptions=Index vector (dialog),Index vector (dialog)  Indices=1,1  OutputSizes=1,1
  11 : Selector  NumberOfDimensions=2  InputPortWidth=3  IndexOptions=Index vector (dialog),Index vector (dialog)  Indices=1,1  OutputSizes=1,1
  12 : Selector  NumberOfDimensions=2  InputPortWidth=3  IndexOptions=Index vector (dialog),Index vector (dialog)  Indices=1,2  OutputSizes=1,1
  2 : Selector  NumberOfDimensions=2  InputPortWidth=3  IndexOptions=Index vector (dialog),Index vector (dialog)  Indices=1,1  OutputSizes=1,1
  Add2 : Sum  Inputs=+++
  Constant1 : Constant  Value=0  VectorParams1D=off
  Constant2 : Constant  Value=0  VectorParams1D=off
  Constant3 : Constant  Value=[0 1]  VectorParams1D=off
  Constant4 : Constant  Value=0  VectorParams1D=off
  Demux2 : Demux  Outputs=2
  Demux3 : Demux  Outputs=2
  Gain : Gain  Gain=-1
  Gain1 : Gain  Gain=-1
  Gain2 : Gain  Gain=-1
  Modelled Plant : Subsystem  TreatAsAtomicUnit=on
  Mux{1..4} (4 alike) : Mux  Inputs=2
  Product{1..2,4..6} (5 alike) : Product  Multiplication=Matrix(*)  RndMeth=Zero
  Product3 : Product  Inputs=/  Multiplication=Matrix(*)  RndMeth=Zero
  Reshape1 : Reshape  OutputDimensionality=Row vector (2-D)
  Reshape2 : Reshape  OutputDimensionality=Column vector (2-D)
  Reshape3 : Reshape  OutputDimensionality=Column vector (2-D)
  Reshape4 : Reshape  OutputDimensionality=Column vector (2-D)
  Terminator : Terminator
  Vector Concatenate : Concatenate  Mode=Multidimensional array
  f1 : Outport
  wires:
  [f1] -> f1/1
  [C] -> 12/1, 11/1
  11/1 -> [C11]
  12/1 -> [C12]
  [G] -> 1/1
  1/1 -> [G1]
  qdot/1 -> [qdot], Demux3/1
  q/1 -> [q], Demux2/1
  Demux3/2 -> [q2dot]
  Demux3/1 -> [q1dot]
  Demux2/2 -> Terminator/1
  Demux2/1 -> [q1]
  [H] -> 2/1
  2/1 -> Product3/1
  Product3/1 -> [H11inv]
  Product1/1 -> Add2/1
  Add2/1 -> [f1]
  [H11inv] -> Product2/1
  [C11] -> Product2/2
  Modelled Plant/1(H) -> [H]
  Modelled Plant/2(C) -> [C]
  Modelled Plant/3(G) -> [G]
  [qdot] -> Modelled Plant/2(qdot)
  [q] -> Modelled Plant/1(q)
  [q1dot] -> Mux1/2
  [q1] -> Mux1/1
  Mux1/1 -> Reshape2/1
  Reshape2/1 -> [x1]
  Product2/1 -> Gain/1
  Constant1/1 -> Mux2/1
  Mux2/1 -> Reshape1/1
  Constant3/1 -> Vector Concatenate/1
  Reshape1/1 -> Vector Concatenate/2
  Vector Concatenate/1 -> [A]
  [A] -> Product1/1
  [x1] -> Product1/2
  [H11inv] -> Product4/1
  [G1] -> Product4/2
  Gain/1 -> Mux2/2
  Product4/1 -> Gain1/1
  Constant2/1 -> Mux3/1
  Mux3/1 -> Reshape3/1
  Gain1/1 -> Mux3/2
  [H11inv] -> Product5/1
  [C12] -> Product5/2
  Constant4/1 -> Mux4/1
  Mux4/1 -> Reshape4/1
  Gain2/1 -> Mux4/2
  Product5/1 -> Product6/1
  [q2dot] -> Product6/2
  Product6/1 -> Gain2/1
  Reshape3/1 -> Add2/2
  Reshape4/1 -> Add2/3

== system simTwoLinkFTC/Controller/FTC Controller/1st Link Compensator/Partial FBL q2 Controller/Collocated q2 Controller ==
  r : Inport
  rdot : Inport  Port=2
  q : Inport  Port=3
  qdot : Inport  Port=4
  Add3 : Sum
  Gain2 : Gain  Gain=-K1
  Gain3 : Gain  Gain=-K2
  sum1 : Sum  Inputs=+-
  sum2 : Sum  Inputs=+-
  v : Outport
  wires:
  Add3/1 -> [v]
  Gain3/1 -> Add3/2
  Gain2/1 -> Add3/1
  [e] -> Gain3/1
  [edot] -> Gain2/1
  qdot/1 -> [qdot]  "qdot"
  q/1 -> [q]  "q"
  [q] -> sum1/1
  [r] -> sum1/2
  sum1/1 -> [e]  "e"
  r/1 -> [r]  "r"
  [v] -> v/1  "v"
  [qdot] -> sum2/1
  [rdot] -> sum2/2
  sum2/1 -> [edot]  "edot"
  rdot/1 -> [rdot]  "rdot"

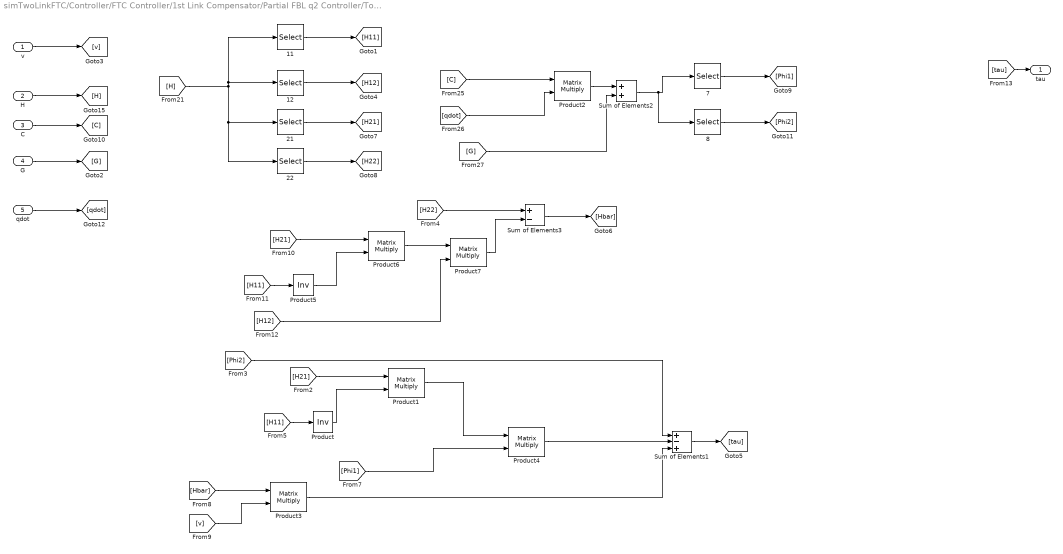
== system simTwoLinkFTC/Controller/FTC Controller/1st Link Compensator/Partial FBL q2 Controller/Torque calculation ==
  v : Inport
  H : Inport  Port=2
  C : Inport  Port=3
  G : Inport  Port=4
  qdot : Inport  Port=5
  11 : Selector  NumberOfDimensions=2  InputPortWidth=3  IndexOptions=Index vector (dialog),Index vector (dialog)  Indices=1,1  OutputSizes=1,1
  12 : Selector  NumberOfDimensions=2  InputPortWidth=3  IndexOptions=Index vector (dialog),Index vector (dialog)  Indices=1,2  OutputSizes=1,1
  21 : Selector  NumberOfDimensions=2  InputPortWidth=3  IndexOptions=Index vector (dialog),Index vector (dialog)  Indices=2,1  OutputSizes=1,1
  22 : Selector  NumberOfDimensions=2  InputPortWidth=3  IndexOptions=Index vector (dialog),Index vector (dialog)  Indices=2,2  OutputSizes=1,1
  7 : Selector  NumberOfDimensions=2  InputPortWidth=3  IndexOptions=Index vector (dialog),Index vector (dialog)  Indices=1,1  OutputSizes=1,1
  8 : Selector  NumberOfDimensions=2  InputPortWidth=3  IndexOptions=Index vector (dialog),Index vector (dialog)  Indices=2,1  OutputSizes=1,1
  Product : Product  Inputs=/  Multiplication=Matrix(*)  RndMeth=Zero
  Product{1..4,6..7} (6 alike) : Product  Multiplication=Matrix(*)  RndMeth=Zero
  Product5 : Product  Inputs=/  Multiplication=Matrix(*)  RndMeth=Zero
  Sum of Elements1 : Sum  Inputs=+-+
  Sum of Elements2 : Sum
  Sum of Elements3 : Sum  Inputs=+-
  tau : Outport
  wires:
  [tau] -> tau/1
  v/1 -> [v]
  [H11] -> Product/1
  [H21] -> Product1/1
  Product/1 -> Product1/2
  Product1/1 -> Product4/1
  [Hbar] -> Product3/1
  [v] -> Product3/2
  Sum of Elements1/1 -> [tau]
  [H11] -> Product5/1
  [H21] -> Product6/1
  Product5/1 -> Product6/2
  Product6/1 -> Product7/1
  [H12] -> Product7/2
  [H22] -> Sum of Elements3/1
  Product7/1 -> Sum of Elements3/2
  Sum of Elements3/1 -> [Hbar]
  [Phi1] -> Product4/2
  [Phi2] -> Sum of Elements1/1
  Product4/1 -> Sum of Elements1/2
  Product3/1 -> Sum of Elements1/3
  C/1 -> [C]
  H/1 -> [H]
  G/1 -> [G]
  [H] -> 11/1, 12/1, 21/1, 22/1
  [C] -> Product2/1
  [qdot] -> Product2/2
  Product2/1 -> Sum of Elements2/1
  [G] -> Sum of Elements2/2
  Sum of Elements2/1 -> 7/1, 8/1
  11/1 -> [H11]
  12/1 -> [H12]
  21/1 -> [H21]
  22/1 -> [H22]
  7/1 -> [Phi1]
  8/1 -> [Phi2]
  qdot/1 -> [qdot]

== system simTwoLinkFTC/Controller/Disturbance Estimator/getDisturbance/Chebyshev Basis Functions/Chebyshev Polynomail Value Calculation/If Action Subsystem ==
  x : Inport
  polyvals : Inport  Port=2
  Action Port : ActionPort  PropagateVarSize=During execution  ActionType=then
  Add : Sum  Inputs=+-
  Constant : Constant  Value=nCheby
  Constant1 : Constant  Value=nCheby-1
  Gain : Gain  Gain=2
  Product : Product  RndMeth=Zero
  Selector : Selector  IndexOptions=Index vector (port)  Indices=[1 3]
  Selector1 : Selector  IndexOptions=Index vector (port)  Indices=[1 3]
  polyval : Outport
  wires:
  x/1 -> [x]
  polyvals/1 -> [polyvals]  "if.polyvals"
  [polyvals] -> Selector/1
  Constant1/1 -> Selector/2
  Selector/1 -> [Tm2]  "Tm2"
  [polyvals] -> Selector1/1
  Constant/1 -> Selector1/2
  Selector1/1 -> [Tm1]  "Tm1"
  [x] -> Product/1
  [Tm1] -> Product/2
  Product/1 -> Gain/1
  Gain/1 -> Add/1
  [Tm2] -> Add/2
  Add/1 -> polyval/1  "if.polyval"

== system simTwoLinkFTC/Controller/Disturbance Estimator/getDisturbance/Chebyshev Basis Functions/Chebyshev Polynomail Value Calculation/If Action Subsystem1 ==
  x : Inport
  N : Inport  Port=2
  Action Port : ActionPort  PropagateVarSize=During execution  ActionType=else
  Bias1 : Bias  Bias=-1
  Data Type Conversion : DataTypeConversion
  Math Function : Math  Operator=pow  OutputSignalType=real  SaturateOnIntegerOverflow=on
  polval : Outport
  wires:
  x/1 -> Math Function/1
  N/1 -> Bias1/1  "else.N"
  Math Function/1 -> polval/1  "else.polyval"
  Data Type Conversion/1 -> Math Function/2
  Bias1/1 -> Data Type Conversion/1

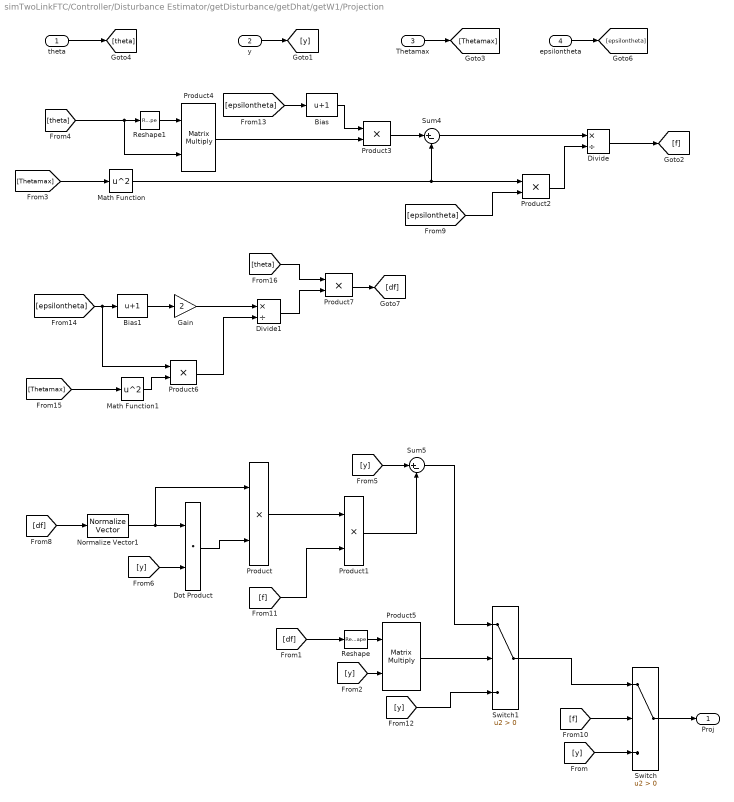
== system simTwoLinkFTC/Controller/Disturbance Estimator/getDisturbance/getDhat/getW1/Projection ==
  theta : Inport
  y : Inport  Port=2
  Thetamax : Inport  Port=3
  epsilontheta : Inport  Port=4
  Bias : Bias  Bias=1
  Bias1 : Bias  Bias=1
  Divide : Product  Inputs=*/
  Divide1 : Product  Inputs=*/
  Dot Product : DotProduct  InputSameDT=on  OutDataTypeStr=Inherit: Inherit via internal rule
  Gain : Gain  Gain=2
  Math Function : Math  Operator=square  SaturateOnIntegerOverflow=on
  Math Function1 : Math  Operator=square  SaturateOnIntegerOverflow=on
  Normalize Vector1 : vrlib/Utilities/Normalize Vector  maxzero=0
  Product{,1..3,6..7} (6 alike) : Product  RndMeth=Zero
  Product4 : Product  Multiplication=Matrix(*)  RndMeth=Zero
  Product5 : Product  Multiplication=Matrix(*)  RndMeth=Zero
  Reshape : Reshape  OutputDimensionality=Row vector (2-D)
  Reshape1 : Reshape  OutputDimensionality=Row vector (2-D)
  Sum4 : Sum  Inputs=|+-
  Sum5 : Sum  Inputs=|+-
  Switch : Switch  Criteria=u2 > Threshold
  Switch1 : Switch  Criteria=u2 > Threshold
  Proj : Outport
  wires:
  [f] -> Switch/2
  y/1 -> [y]
  Switch/1 -> Proj/1
  Product5/1 -> Switch1/2
  [y] -> Product5/2
  Sum4/1 -> Divide/1
  Math Function/1 -> Sum4/2, Product2/1
  Product4/1 -> Product3/2
  [theta] -> Reshape1/1, Product4/2
  [df] -> Reshape/1
  Reshape/1 -> Product5/1
  Reshape1/1 -> Product4/1
  theta/1 -> [theta]
  [y] -> Switch/3
  Switch1/1 -> Switch/1
  [y] -> Sum5/1
  Product/1 -> Product1/1
  [y] -> Switch1/3
  Product1/1 -> Sum5/2
  Sum5/1 -> Switch1/1
  [f] -> Product1/2
  [df] -> Normalize Vector1/1
  Normalize Vector1/1 -> Dot Product/1, Product/1
  [y] -> Dot Product/2
  Dot Product/1 -> Product/2
  Thetamax/1 -> [Thetamax]
  [Thetamax] -> Math Function/1
  epsilontheta/1 -> [epsilontheta]
  [epsilontheta] -> Product2/2
  Product2/1 -> Divide/2
  Divide/1 -> [f]
  Product3/1 -> Sum4/1
  Bias/1 -> Product3/1
  [epsilontheta] -> Bias/1
  [epsilontheta] -> Bias1/1, Product6/1
  Bias1/1 -> Gain/1
  Gain/1 -> Divide1/1
  [Thetamax] -> Math Function1/1
  Math Function1/1 -> Product6/2
  Product6/1 -> Divide1/2
  Product7/1 -> [df]
  [theta] -> Product7/1
  Divide1/1 -> Product7/2

== system simTwoLinkFTC/Controller/Disturbance Estimator/getDisturbance/getDhat/getW2/Projection ==
  theta : Inport
  y : Inport  Port=2
  Thetamax : Inport  Port=3
  epsilontheta : Inport  Port=4
  Bias : Bias  Bias=1
  Bias1 : Bias  Bias=1
  Divide : Product  Inputs=*/
  Divide1 : Product  Inputs=*/
  Dot Product : DotProduct  InputSameDT=on  OutDataTypeStr=Inherit: Inherit via internal rule
  Gain : Gain  Gain=2
  Math Function : Math  Operator=square  SaturateOnIntegerOverflow=on
  Math Function1 : Math  Operator=square  SaturateOnIntegerOverflow=on
  Normalize Vector1 : vrlib/Utilities/Normalize Vector  maxzero=0
  Product{,1..3,6..7} (6 alike) : Product  RndMeth=Zero
  Product4 : Product  Multiplication=Matrix(*)  RndMeth=Zero
  Product5 : Product  Multiplication=Matrix(*)  RndMeth=Zero
  Reshape : Reshape  OutputDimensionality=Row vector (2-D)
  Reshape1 : Reshape  OutputDimensionality=Row vector (2-D)
  Sum4 : Sum  Inputs=|+-
  Sum5 : Sum  Inputs=|+-
  Switch : Switch  Criteria=u2 > Threshold
  Switch1 : Switch  Criteria=u2 > Threshold
  Proj : Outport
  wires:
  Divide1/1 -> Product7/2
  [theta] -> Product7/1
  Product7/1 -> [df]
  Product6/1 -> Divide1/2
  Math Function1/1 -> Product6/2
  [Thetamax] -> Math Function1/1
  Gain/1 -> Divide1/1
  Bias1/1 -> Gain/1
  [epsilontheta] -> Product6/1, Bias1/1
  [epsilontheta] -> Bias/1
  Bias/1 -> Product3/1
  Product3/1 -> Sum4/1
  Divide/1 -> [f]
  Product2/1 -> Divide/2
  [epsilontheta] -> Product2/2
  epsilontheta/1 -> [epsilontheta]
  [Thetamax] -> Math Function/1
  Thetamax/1 -> [Thetamax]
  Dot Product/1 -> Product/2
  [y] -> Dot Product/2
  Normalize Vector1/1 -> Product/1, Dot Product/1
  [df] -> Normalize Vector1/1
  [f] -> Product1/2
  Sum5/1 -> Switch1/1
  Product1/1 -> Sum5/2
  [y] -> Switch1/3
  Product/1 -> Product1/1
  [y] -> Sum5/1
  Switch1/1 -> Switch/1
  [y] -> Switch/3
  theta/1 -> [theta]
  Reshape1/1 -> Product4/1
  Reshape/1 -> Product5/1
  [df] -> Reshape/1
  [theta] -> Product4/2, Reshape1/1
  Product4/1 -> Product3/2
  Math Function/1 -> Product2/1, Sum4/2
  Sum4/1 -> Divide/1
  [y] -> Product5/2
  Product5/1 -> Switch1/2
  Switch/1 -> Proj/1
  y/1 -> [y]
  [f] -> Switch/2

== system simTwoLinkFTC/Controller/FTC Controller/1st Link Compensator/ ADI Controller/System model/Modelled Plant ==
  q : Inport
  qdot : Inport  Port=2
  Demux : Demux  Outputs=2
  Demux1 : Demux  Outputs=2
  Demux2 : Demux  Outputs=2
  Sum of Elements : Sum  Inputs=+
  Terminator4 : Terminator
  Terminator5 : Terminator
  Terminator6 : Terminator
  Trigonometric Function : Trigonometry
  Trigonometric Function1 : Trigonometry  Operator=cos
  Trigonometric Function2 : Trigonometry
  Trigonometric Function3 : Trigonometry  Operator=cos
  get Plant Parameters : Subsystem
  getC : Subsystem
  getG : Subsystem
  getH : Subsystem
  H : Outport
  C : Outport  Port=2
  G : Outport  Port=3
  wires:
  [c2] -> getH/1(c2)
  [s2] -> getC/1(s2)
  [q1dot] -> getC/2(q1dot)
  [q2dot] -> getC/3(q2dot)
  getH/1(H) -> [H]
  getC/1(C) -> [C]
  [c1] -> getG/1(c1)
  [c12] -> getG/2(c12)
  getG/1(G) -> [G]
  q/1 -> Trigonometric Function/1, Trigonometric Function1/1, Sum of Elements/1
  Trigonometric Function/1 -> Demux/1
  Demux/1 -> Terminator4/1
  Demux/2 -> [s2]
  Demux1/1 -> [c1]
  Demux1/2 -> [c2]
  Trigonometric Function1/1 -> Demux1/1
  Sum of Elements/1 -> Trigonometric Function2/1, Trigonometric Function3/1
  Trigonometric Function2/1 -> Terminator5/1
  qdot/1 -> Demux2/1, [qdot]
  Demux2/1 -> [q1dot]
  Demux2/2 -> [q2dot]
  Trigonometric Function3/1 -> [c12]
  [H] -> H/1
  [C] -> C/1
  [G] -> G/1
  get Plant Parameters/1(busData) -> Terminator6/1  "ModeledSystem"
  [C] -> get Plant Parameters/2(C)
  [H] -> get Plant Parameters/1(H)
  [G] -> get Plant Parameters/3(G)
  [qdot] -> get Plant Parameters/4(qdot)

== system simTwoLinkFTC/Controller/FTC Controller/1st Link Compensator/ ADI Controller/System model/Modelled Plant/get Plant Parameters ==
  H : Inport
  C : Inport  Port=2
  G : Inport  Port=3
  qdot : Inport  Port=4
  {1,5,7,11} (4 alike) : Selector  NumberOfDimensions=2  InputPortWidth=3  IndexOptions=Index vector (dialog),Index vector (dialog)  Indices=1,1  OutputSizes=1,1
  12 : Selector  NumberOfDimensions=2  InputPortWidth=3  IndexOptions=Index vector (dialog),Index vector (dialog)  Indices=1,2  OutputSizes=1,1
  2 : Selector  NumberOfDimensions=2  InputPortWidth=3  IndexOptions=Index vector (dialog),Index vector (dialog)  Indices=1,2  OutputSizes=1,1
  {3,6,8,21} (4 alike) : Selector  NumberOfDimensions=2  InputPortWidth=3  IndexOptions=Index vector (dialog),Index vector (dialog)  Indices=2,1  OutputSizes=1,1
  22 : Selector  NumberOfDimensions=2  InputPortWidth=3  IndexOptions=Index vector (dialog),Index vector (dialog)  Indices=2,2  OutputSizes=1,1
  4 : Selector  NumberOfDimensions=2  InputPortWidth=3  IndexOptions=Index vector (dialog),Index vector (dialog)  Indices=2,2  OutputSizes=1,1
  Bus Creator : BusCreator  Inputs=15
  Product5 : Product  Multiplication=Matrix(*)  RndMeth=Zero
  Sum of Elements1 : Sum
  busData : Outport
  wires:
  2/1 -> Bus Creator/9  "C12"
  21/1 -> Bus Creator/6  "H21"
  22/1 -> Bus Creator/7  "H22"
  4/1 -> Bus Creator/11  "C22"
  6/1 -> Bus Creator/13  "G_2"
  1/1 -> Bus Creator/8  "C11"
  5/1 -> Bus Creator/12  "G_1"
  12/1 -> Bus Creator/5  "H12"
  3/1 -> Bus Creator/10  "C21"
  11/1 -> Bus Creator/4  "H11"
  [H] -> 11/1, 12/1, 21/1, 22/1
  [C] -> 1/1, 2/1, 4/1, 3/1
  [G] -> 6/1, 5/1
  [C] -> Product5/1
  [qdot] -> Product5/2
  Product5/1 -> Sum of Elements1/1
  [G] -> Sum of Elements1/2
  Sum of Elements1/1 -> 7/1, 8/1
  7/1 -> Bus Creator/14  "phi1"
  8/1 -> Bus Creator/15  "phi2"
  [G] -> Bus Creator/3
  Bus Creator/1 -> busData/1
  [C] -> Bus Creator/2
  [H] -> Bus Creator/1
  H/1 -> [H]  "H"
  C/1 -> [C]  "C"
  G/1 -> [G]  "G"
  qdot/1 -> [qdot]

== system simTwoLinkFTC/Controller/FTC Controller/1st Link Compensator/ ADI Controller/System model/Modelled Plant/getC ==
  s2 : Inport
  q1dot : Inport  Port=2
  q2dot : Inport  Port=3
  C calculation 1 : Subsystem
  C calculation 2 : Subsystem
  Gain2 : Gain  Gain=m2*l1*lc2
  Terminator : Terminator
  C : Outport
  wires:
  s2/1 -> [s2]
  q1dot/1 -> [q1dot]
  q2dot/1 -> [q2dot]
  [s2] -> Gain2/1
  Gain2/1 -> [h]
  [q1dot] -> C calculation 1/1(q1dot)
  [q2dot] -> C calculation 1/2(q2dot)
  [h] -> C calculation 1/3(h)
  [q1dot] -> C calculation 2/1(q1dot)
  [q2dot] -> C calculation 2/2(q2dot)
  [h] -> C calculation 2/3(h)
  [C] -> C/1
  C calculation 2/1(C) -> [C]
  C calculation 1/1(C) -> Terminator/1

== system simTwoLinkFTC/Controller/FTC Controller/1st Link Compensator/ ADI Controller/System model/Modelled Plant/getG ==
  c1 : Inport
  c12 : Inport  Port=2
  Add : Sum
  Gain : Gain  Gain=(m1*lc1+m2*l1)*g
  Gain1 : Gain  Gain=m2*g*lc2
  Gain2 : Gain
  Gain4 : Gain  Gain=lc2*m2*g
  Matrix Concatenate2 : Concatenate  Mode=Multidimensional array
  G : Outport
  wires:
  [c12] -> Gain4/1
  Gain4/1 -> [G21]
  c12/1 -> [c12]
  c1/1 -> [c1]
  Matrix Concatenate2/1 -> Gain2/1
  [G11] -> Matrix Concatenate2/1
  [G21] -> Matrix Concatenate2/2
  [c1] -> Gain/1
  Gain/1 -> Add/1
  [c12] -> Gain1/1
  Gain1/1 -> Add/2
  Add/1 -> [G11]
  Gain2/1 -> G/1

== system simTwoLinkFTC/Controller/FTC Controller/1st Link Compensator/ ADI Controller/System model/Modelled Plant/getH ==
  c2 : Inport
  Constant1 : Constant  Value=I1 + I2 + m1*lc1^2 + m2*(l1^2+lc2^2)  VectorParams1D=off
  Constant2 : Constant  Value=I2+m2*lc2^2  VectorParams1D=off
  Constant3 : Constant  Value=I2+m2*lc2^2  VectorParams1D=off
  Gain : Gain  Gain=m2*2*l1*lc2
  Gain1 : Gain  Gain=m2*l1*lc2
  Matrix Concatenate : Concatenate  Mode=Multidimensional array  ConcatenateDimension=2
  Matrix Concatenate1 : Concatenate  Mode=Multidimensional array  ConcatenateDimension=2
  Matrix Concatenate2 : Concatenate  Mode=Multidimensional array
  Sum : Sum
  Sum1 : Sum
  H : Outport
  wires:
  [H11] -> Matrix Concatenate/1
  [H12] -> Matrix Concatenate/2
  Matrix Concatenate/1 -> Matrix Concatenate2/1
  Matrix Concatenate1/1 -> Matrix Concatenate2/2
  [H21] -> Matrix Concatenate1/1
  [H22] -> Matrix Concatenate1/2
  Matrix Concatenate2/1 -> H/1
  c2/1 -> [c2]
  [c2] -> Gain/1
  Gain/1 -> Sum/1
  Constant1/1 -> Sum/2
  Sum/1 -> [H11]
  [c2] -> Gain1/1
  Gain1/1 -> Sum1/1
  Constant2/1 -> Sum1/2
  Sum1/1 -> [H12], [H21]
  Constant3/1 -> [H22]

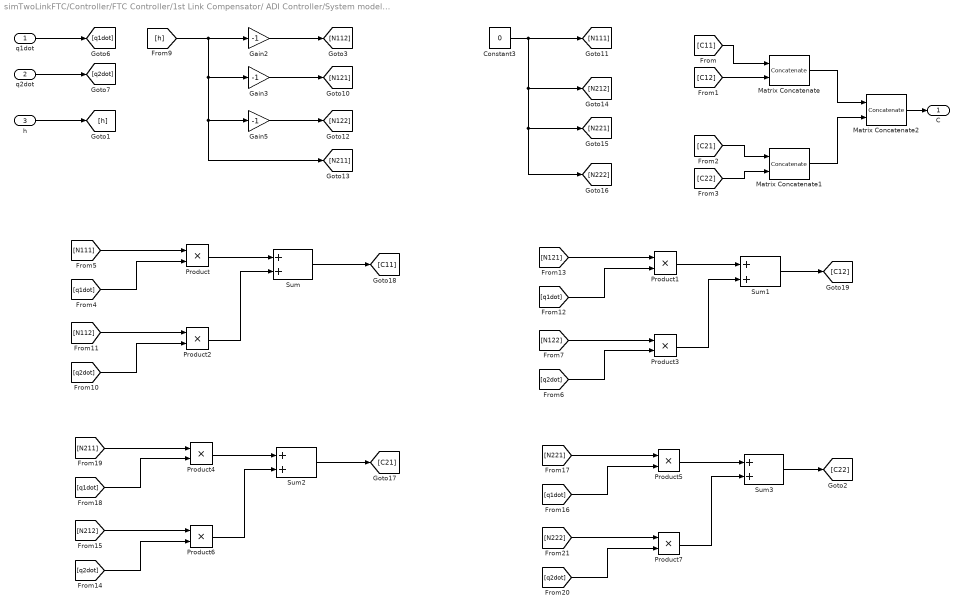
== system simTwoLinkFTC/Controller/FTC Controller/1st Link Compensator/ ADI Controller/System model/Modelled Plant/getC/C calculation 1 ==
  q1dot : Inport
  q2dot : Inport  Port=2
  h : Inport  Port=3
  Constant3 : Constant  Value=0  VectorParams1D=off
  Gain2 : Gain  Gain=-1
  Gain3 : Gain  Gain=-1
  Gain5 : Gain  Gain=-1
  Matrix Concatenate : Concatenate  Mode=Multidimensional array  ConcatenateDimension=2
  Matrix Concatenate1 : Concatenate  Mode=Multidimensional array  ConcatenateDimension=2
  Matrix Concatenate2 : Concatenate  Mode=Multidimensional array
  Product{,1..7} (8 alike) : Product  RndMeth=Zero
  Sum{,1..3} (4 alike) : Sum
  C : Outport
  wires:
  q2dot/1 -> [q2dot]
  q1dot/1 -> [q1dot]
  [N111] -> Product/1
  Product/1 -> Sum/1
  [q1dot] -> Product/2
  [N112] -> Product2/1
  Product2/1 -> Sum/2
  [q2dot] -> Product2/2
  Sum/1 -> [C11]
  [N121] -> Product1/1
  Product1/1 -> Sum1/1
  [q1dot] -> Product1/2
  [N122] -> Product3/1
  Product3/1 -> Sum1/2
  [q2dot] -> Product3/2
  Sum1/1 -> [C12]
  [N211] -> Product4/1
  Product4/1 -> Sum2/1
  [q1dot] -> Product4/2
  [N212] -> Product6/1
  Product6/1 -> Sum2/2
  [q2dot] -> Product6/2
  Sum2/1 -> [C21]
  [N221] -> Product5/1
  Product5/1 -> Sum3/1
  [q1dot] -> Product5/2
  [N222] -> Product7/1
  Product7/1 -> Sum3/2
  [q2dot] -> Product7/2
  Constant3/1 -> [N111], [N212], [N221], [N222]
  [h] -> Gain2/1, Gain3/1, Gain5/1, [N211]
  Gain2/1 -> [N112]
  Gain3/1 -> [N121]
  Gain5/1 -> [N122]
  h/1 -> [h]
  Sum3/1 -> [C22]
  Matrix Concatenate2/1 -> C/1
  [C22] -> Matrix Concatenate1/2
  [C21] -> Matrix Concatenate1/1
  Matrix Concatenate1/1 -> Matrix Concatenate2/2
  Matrix Concatenate/1 -> Matrix Concatenate2/1
  [C12] -> Matrix Concatenate/2
  [C11] -> Matrix Concatenate/1

== system simTwoLinkFTC/Controller/FTC Controller/1st Link Compensator/ ADI Controller/System model/Modelled Plant/getC/C calculation 2 ==
  q1dot : Inport
  q2dot : Inport  Port=2
  h : Inport  Port=3
  Constant1 : Constant  Value=0  VectorParams1D=off
  Gain6 : Gain  Gain=-2
  Gain7 : Gain  Gain=-1
  Matrix Concatenate : Concatenate  Mode=Multidimensional array  ConcatenateDimension=2
  Matrix Concatenate1 : Concatenate  Mode=Multidimensional array  ConcatenateDimension=2
  Matrix Concatenate2 : Concatenate  Mode=Multidimensional array
  Product10 : Product  RndMeth=Zero
  Product8 : Product  RndMeth=Zero
  Product9 : Product  RndMeth=Zero
  C : Outport
  wires:
  h/1 -> [h]
  q1dot/1 -> [q1dot]
  q2dot/1 -> [q2dot]
  [h] -> Gain6/1
  [h] -> Gain7/1
  Gain7/1 -> Product10/2
  Product10/1 -> [C12]
  Constant1/1 -> [C22]
  [h] -> Product8/2
  [q1dot] -> Product8/1
  Product8/1 -> [C21]
  Gain6/1 -> Product9/2
  Product9/1 -> [C11]
  [q2dot] -> Product9/1
  Matrix Concatenate2/1 -> C/1
  [C22] -> Matrix Concatenate1/2
  [C21] -> Matrix Concatenate1/1
  Matrix Concatenate1/1 -> Matrix Concatenate2/2
  Matrix Concatenate/1 -> Matrix Concatenate2/1
  [C12] -> Matrix Concatenate/2
  [C11] -> Matrix Concatenate/1
  [q2dot] -> Product10/1
